simulink subsystem "PvtSubSys_LATC"  (R2020b)
settings: Solver=VariableStepAuto  StartTime=0.0  StopTime=10.0  RelTol=1e-3
undefined symbols (not defined in the file or in its folder): LCS_PLAN_PreViewIdxNum, LCS_PLAN_PreViewIdxSW_b, P_Global_CharSpd_ms, P_Global_SteeringAngleRatio, P_Global_WheelBase_m, P_LCS_DetNoOverRide_DrvTrq_TH, P_LCS_DetOverRide_DrvTrq_TH, P_LCS_ESS_AngleSlope_Limit, P_LCS_ESS_LogicTest_Enable, P_LCS_ESS_NotActiveFlgDelayTime, P_LCS_ESS_NotActiveFlgDelayTimeSW, P_LCS_ESS_SteerAngleErr, P_LCS_ESS_SteerAngleFilterTime, P_LCS_ESS_TarAngleFilterTime, P_LCS_ESSAngleSW, P_LCS_ESSOverrideTime1, P_LCS_ESSOverrideTime2, P_LCS_ESSOverrideTime3, P_LCS_ESSOverrideValue1, P_LCS_ESSOverrideValue2, P_LCS_IN_Offset_Test_SW, P_LCS_IN_Offset_Test_Value, P_LCS_LATC_AngleFilterTime_s, P_LCS_LATC_CurOffsetCurve_TabX_m, P_LCS_LATC_CurOffsetCurveFliterTime_Tab_s, P_LCS_LATC_CurOffsetVehicleSpdLimitValue_degs, P_LCS_LATC_DeltaEps_Tab_s, P_LCS_LATC_DxOffset_Sw, P_LCS_LATC_ELKAngleSlope_ratio, P_LCS_LATC_ELKMaxLatAcc_ms2, P_LCS_LATC_ESSA0Dis_TabX_m, P_LCS_LATC_ESSAddAngleSlope_Tab_degs, P_LCS_LATC_ESSAESAngleSlope_Tab_degs, P_LCS_LATC_ESSAngleSlope_ratio, P_LCS_LATC_ESSMaxLatAcc_ms2, P_LCS_LATC_LCAngleSlope_ratio, P_LCS_LATC_LCAngleSlope_Tab_degs, P_LCS_LATC_LCCancleMaxLatAcc_ms2, P_LCS_LATC_LCEcoAngleSlope_ratio, P_LCS_LATC_LCEcoAngleSlope_Tab_degs, P_LCS_LATC_LCEcoMaxLatAcc_ms2, P_LCS_LATC_LCKAngleSlope_ratio, P_LCS_LATC_LCKAngleSlope_Tab_degs, P_LCS_LATC_LCKIEAngleSlope_ratio, P_LCS_LATC_LCKIEAngleSlope_Tab_degs, P_LCS_LATC_LCKIEMaxLatAcc_ms2, P_LCS_LATC_LCKMaxLatAcc_ms2, P_LCS_LATC_LCNormalAngleSlope_ratio, P_LCS_LATC_LCNormalAngleSlope_Tab_degs, P_LCS_LATC_LCNormalMaxLatAcc_ms2, P_LCS_LATC_LCSportAngleSlope_ratio, P_LCS_LATC_LCSportAngleSlope_Tab_degs, P_LCS_LATC_LCSportMaxLatAcc_ms2, P_LCS_LATC_LKAAngleSlope_ratio, P_LCS_LATC_LKAAngleSlope_Tab_degs, P_LCS_LATC_LKAMaxLatAcc_ms2, P_LCS_LATC_MatrixQ1_st, P_LCS_LATC_MatrixQ3_st, P_LCS_LATC_MatrixR_st, P_LCS_LATC_MPCDeltaT_s ... (+70)
libraries: simulink x34
(part 4 of 5)

== system PvtSubSys_LATC/Subsystem/LateralControl/LCS_Angle/Lateral_Control/Dynamic_Model_LQR/SteerAngSlopeCalc/Switch Case Action Subsystem ==
  Flg : Inport
  StateHoldTime : Inport  Port=2
  Action Port : ActionPort
  LC_start_slope : Lookup_n-D  BreakpointsForDimension1=P_LCS_LATC_StateActiveFlg_TabX_st  BreakpointsForDimension2=P_LCS_LATC_StateActiveHoldTime_TabY_st  Table=P_LCS_LATC_StateActivAngleSlopeLimit_ratio  ExtrapMethod=Clip  UseLastTableValue=on  InternalRulePriority=Speed  OutDataTypeStr=single  RndMeth=Simplest
      settings: InputPortMap=u0,u1
  Out1 : Outport
  wires:
  Flg/1 -> LC_start_slope/1
  LC_start_slope/1 -> Out1/1
  StateHoldTime/1 -> LC_start_slope/2

== system PvtSubSys_LATC/Subsystem/LateralControl/LCS_Angle/Lateral_Control/Dynamic_Model_LQR/SteerAngSlopeCalc/Switch Case Action Subsystem1 ==
  Action Port : ActionPort
  Constant : Constant  Value=100  OutDataTypeStr=single
  Out1 : Outport
  wires:
  Constant/1 -> Out1/1

== system PvtSubSys_LATC/Subsystem/LateralControl/LCS_Angle/Lateral_Control/Dynamic_Model_LQR/Understeer&Offset_Calc/Enabled Subsystem ==
  AckConst : Inport
  Raw : Inport  Port=2
  Curve : Inport  Port=3
  Enable : EnablePort
  Constant2 : Constant  Value=0.02  OutDataTypeStr=single
  Constant7 : Constant  Value=P_Global_SteeringAngleRatio
  Constant8 : Constant  Value=57.3  OutDataTypeStr=single
  FilterTime2 : Product  Inputs=4  RndMeth=Zero
  Product2 : Product  Inputs=*/  RndMeth=Zero
  Product6 : Product  RndMeth=Zero
  Sum6 : Sum  Inputs=+-
  Sum7 : Sum
  Unit Delay : UnitDelay  SampleTime=-1  HasFrameUpgradeWarning=on
  predis_ayFac1 : Lookup_n-D  NumberOfTableDimensions=1  BreakpointsForDimension1=P_LCS_LATC_CurOffsetCurve_TabX_m  Table=P_LCS_LATC_CurOffsetCurveFliterTime_Tab_s  ExtrapMethod=Clip  UseLastTableValue=on  InternalRulePriority=Speed  RndMeth=Simplest  InputSameDT=on
  SteerAngleOffset_deg : Outport
  wires:
  Sum7/1 -> SteerAngleOffset_deg/1, Unit Delay/1
  Unit Delay/1 -> Sum6/2, Sum7/2
  Constant2/1 -> Product2/1
  Sum6/1 -> Product6/2
  Product2/1 -> Product6/1
  Product6/1 -> Sum7/1
  Constant7/1 -> FilterTime2/1
  Constant8/1 -> FilterTime2/2
  AckConst/1 -> FilterTime2/3
  Raw/1 -> FilterTime2/4
  FilterTime2/1 -> Sum6/1
  Curve/1 -> predis_ayFac1/1
  predis_ayFac1/1 -> Product2/2

== system PvtSubSys_LATC/Subsystem/LateralControl/LCS_Angle/Lateral_Control/MPC/TargetSteerAngleCalc/LP filter ==
  Raw : Inport
  TorqFilterTime : Inport  Port=2
  Product1 : Product  RndMeth=Zero
  Product4 : Product  Inputs=*/  RndMeth=Zero
  Sum4 : Sum  Inputs=+-|
  Sum5 : Sum
  Unit Delay : UnitDelay  SampleTime=-1  HasFrameUpgradeWarning=on
  Weight/N3 : Constant  Value=0.02  OutDataTypeStr=single
  output : Outport
  wires:
  Sum5/1 -> output/1, Unit Delay/1
  Unit Delay/1 -> Sum5/2, Sum4/2
  Sum4/1 -> Product1/2
  Product1/1 -> Sum5/1
  Raw/1 -> Sum4/1
  Weight/N3/1 -> Product4/1
  Product4/1 -> Product1/1
  TorqFilterTime/1 -> Product4/2

== system PvtSubSys_LATC/Subsystem/LateralControl/LCS_Angle/Lateral_Control/MPC/TargetSteerAngleCalc/LP filter1 ==
  Raw : Inport
  TorqFilterTime : Inport  Port=2
  Memory2 : Memory  InheritSampleTime=on
  Product1 : Product  RndMeth=Zero
  Product4 : Product  Inputs=*/  RndMeth=Zero
  Sum4 : Sum  Inputs=+-|
  Sum5 : Sum  Inputs=++|
  Weight/N3 : Constant  Value=0.02  OutDataTypeStr=single
  output : Outport
  wires:
  TorqFilterTime/1 -> Product4/2
  Product4/1 -> Product1/1
  Weight/N3/1 -> Product4/1
  Raw/1 -> Sum4/1
  Product1/1 -> Sum5/1
  Sum4/1 -> Product1/2
  Memory2/1 -> Sum4/2, Sum5/2
  Sum5/1 -> output/1, Memory2/1

== system PvtSubSys_LATC/Subsystem/LateralControl/LCS_Angle/Lateral_Control/MPC/TargetSteerAngleCalc/Subsystem ==
  Flg : Inport
  HoldTime : Inport  Port=2
  Merge : Merge
  Merge1 : Merge
  Merge2 : Merge
  Switch Case : SwitchCase  CaseConditions={[1,2,3,4,5]}
  Switch Case Action Subsystem : Subsystem  TreatAsAtomicUnit=on
  Switch Case Action Subsystem1 : Subsystem  TreatAsAtomicUnit=on
  Switch Case Action Subsystem2 : Subsystem  TreatAsAtomicUnit=on
  Switch Case Action Subsystem3 : Subsystem  TreatAsAtomicUnit=on
  Switch Case Action Subsystem4 : Subsystem  TreatAsAtomicUnit=on
  Switch Case Action Subsystem5 : Subsystem  TreatAsAtomicUnit=on
  Switch Case1 : SwitchCase  CaseConditions={[6,7,8]}
  Switch Case2 : SwitchCase  CaseConditions={[6,7,8]}
  LC_Complete_AngleSlope : Outport
  LC_Complete_PreDisFac : Outport  Port=2
  StateActiv_AngleSlope : Outport  Port=3
  wires:
  [HoldTime] -> Switch Case Action Subsystem2/2(StateHoldTime)
  Switch Case/2 -> Switch Case Action Subsystem1/Action
  Switch Case Action Subsystem4/1(Out1) -> Merge2/1
  Switch Case Action Subsystem1/1(Out1) -> Merge/1
  Switch Case Action Subsystem3/1(Out1) -> Merge1/1
  Switch Case2/2 -> Switch Case Action Subsystem4/Action
  HoldTime/1 -> Switch Case Action Subsystem5/2(StateHoldTime)
  Flg/1 -> Switch Case/1, Switch Case1/1, Switch Case Action Subsystem5/1(Flg), Switch Case2/1, Switch Case Action Subsystem2/1(Flg), Switch Case Action Subsystem/1(Flg)
  Switch Case2/1 -> Switch Case Action Subsystem5/Action
  Switch Case1/2 -> Switch Case Action Subsystem3/Action
  Switch Case1/1 -> Switch Case Action Subsystem2/Action
  Switch Case Action Subsystem/1(Out1) -> Merge/2
  Switch Case Action Subsystem2/1(Out1) -> Merge1/2
  Switch Case Action Subsystem5/1(LC_Complete_PreDisFac) -> Merge2/2
  Merge2/1 -> LC_Complete_PreDisFac/1
  [HoldTime] -> Switch Case Action Subsystem/2(StateHoldTime)
  Switch Case/1 -> Switch Case Action Subsystem/Action
  Merge1/1 -> LC_Complete_AngleSlope/1
  Merge/1 -> StateActiv_AngleSlope/1

== system PvtSubSys_LATC/Subsystem/LateralControl/LCS_Angle/Lateral_Control/MPC/Understeer_Offset_Calc/Enabled Subsystem ==
  AckConst : Inport
  Raw : Inport  Port=2
  Curve : Inport  Port=3
  Enable : EnablePort
  Constant2 : Constant  Value=0.02  OutDataTypeStr=single
  Constant7 : Constant  Value=P_Global_SteeringAngleRatio
  Constant8 : Constant  Value=57.3  OutDataTypeStr=single
  FilterTime2 : Product  Inputs=4  RndMeth=Zero
  Product2 : Product  Inputs=*/  RndMeth=Zero
  Product6 : Product  RndMeth=Zero
  Sum6 : Sum  Inputs=+-
  Sum7 : Sum
  Unit Delay : UnitDelay  SampleTime=-1  HasFrameUpgradeWarning=on
  predis_ayFac1 : Lookup_n-D  NumberOfTableDimensions=1  BreakpointsForDimension1=P_LCS_LATC_CurOffsetCurve_TabX_m  Table=P_LCS_LATC_CurOffsetCurveFliterTime_Tab_s  ExtrapMethod=Clip  UseLastTableValue=on  InternalRulePriority=Speed  RndMeth=Simplest  InputSameDT=on
  SteerAngleOffset_deg : Outport
  wires:
  Sum7/1 -> SteerAngleOffset_deg/1, Unit Delay/1
  Unit Delay/1 -> Sum6/2, Sum7/2
  Constant2/1 -> Product2/1
  Sum6/1 -> Product6/2
  Product2/1 -> Product6/1
  Product6/1 -> Sum7/1
  Constant7/1 -> FilterTime2/1
  Constant8/1 -> FilterTime2/2
  AckConst/1 -> FilterTime2/3
  Raw/1 -> FilterTime2/4
  FilterTime2/1 -> Sum6/1
  Curve/1 -> predis_ayFac1/1
  predis_ayFac1/1 -> Product2/2

== system PvtSubSys_LATC/Subsystem/LateralControl/LCS_Angle/Lateral_Control/kinematics_MPC/SteerAngSlopeCalc/Switch Case Action Subsystem ==
  Flg : Inport
  StateHoldTime : Inport  Port=2
  Action Port : ActionPort
  LC_start_slope : Lookup_n-D  BreakpointsForDimension1=P_LCS_LATC_StateActiveFlg_TabX_st  BreakpointsForDimension2=P_LCS_LATC_StateActiveHoldTime_TabY_st  Table=P_LCS_LATC_StateActivAngleSlopeLimit_ratio  ExtrapMethod=Clip  UseLastTableValue=on  InternalRulePriority=Speed  OutDataTypeStr=single  RndMeth=Simplest
      settings: InputPortMap=u0,u1
  Out1 : Outport
  wires:
  Flg/1 -> LC_start_slope/1
  LC_start_slope/1 -> Out1/1
  StateHoldTime/1 -> LC_start_slope/2

== system PvtSubSys_LATC/Subsystem/LateralControl/LCS_Angle/Lateral_Control/kinematics_MPC/SteerAngSlopeCalc/Switch Case Action Subsystem1 ==
  Action Port : ActionPort
  Constant : Constant  Value=100  OutDataTypeStr=single
  Out1 : Outport
  wires:
  Constant/1 -> Out1/1

== system PvtSubSys_LATC/Subsystem/LateralControl/LCS_Angle/Lateral_Control/kinematics_MPC/Understeer&Offset_Calc/Enabled Subsystem ==
  AckConst : Inport
  Raw : Inport  Port=2
  Curve : Inport  Port=3
  Enable : EnablePort
  Constant2 : Constant  Value=0.02  OutDataTypeStr=single
  Constant7 : Constant  Value=P_Global_SteeringAngleRatio
  Constant8 : Constant  Value=57.3  OutDataTypeStr=single
  FilterTime2 : Product  Inputs=4  RndMeth=Zero
  Product2 : Product  Inputs=*/  RndMeth=Zero
  Product6 : Product  RndMeth=Zero
  Sum6 : Sum  Inputs=+-
  Sum7 : Sum
  Unit Delay : UnitDelay  SampleTime=-1  HasFrameUpgradeWarning=on
  predis_ayFac1 : Lookup_n-D  NumberOfTableDimensions=1  BreakpointsForDimension1=P_LCS_LATC_CurOffsetCurve_TabX_m  Table=P_LCS_LATC_CurOffsetCurveFliterTime_Tab_s  ExtrapMethod=Clip  UseLastTableValue=on  InternalRulePriority=Speed  RndMeth=Simplest  InputSameDT=on
  SteerAngleOffset_deg : Outport
  wires:
  Sum7/1 -> SteerAngleOffset_deg/1, Unit Delay/1
  Unit Delay/1 -> Sum6/2, Sum7/2
  Constant2/1 -> Product2/1
  Sum6/1 -> Product6/2
  Product2/1 -> Product6/1
  Product6/1 -> Sum7/1
  Constant7/1 -> FilterTime2/1
  Constant8/1 -> FilterTime2/2
  AckConst/1 -> FilterTime2/3
  Raw/1 -> FilterTime2/4
  FilterTime2/1 -> Sum6/1
  Curve/1 -> predis_ayFac1/1
  predis_ayFac1/1 -> Product2/2

== system PvtSubSys_LATC/Subsystem/LateralControl/LCS_Angle/Motion_Planning/CartesianTrajectory/Subsystem1/LP filter ==
  Raw : Inport
  TorqFilterTime : Inport  Port=2
  Product1 : Product  RndMeth=Zero
  Product4 : Product  Inputs=*/  RndMeth=Zero
  Sum4 : Sum  Inputs=+-
  Sum5 : Sum
  Unit Delay : UnitDelay  SampleTime=-1  HasFrameUpgradeWarning=on
  Weight/N3 : Constant  Value=0.02  OutDataTypeStr=single
  output : Outport
  wires:
  Sum5/1 -> output/1, Unit Delay/1
  Unit Delay/1 -> Sum5/2, Sum4/2
  Sum4/1 -> Product1/2
  Product1/1 -> Sum5/1
  Raw/1 -> Sum4/1
  Weight/N3/1 -> Product4/1
  Product4/1 -> Product1/1
  TorqFilterTime/1 -> Product4/2

== system PvtSubSys_LATC/Subsystem/LateralControl/LCS_Angle/Motion_Planning/CartesianTrajectory/Subsystem1/Switch Case Action Subsystem ==
  Flg : Inport
  StateHoldTime : Inport  Port=2
  Action Port : ActionPort
  ActiveAyDtLimit_TBL : Lookup_n-D  BreakpointsForDimension1=P_LCS_LATC_StateActiveFlg_TabX_st  BreakpointsForDimension2=P_LCS_LATC_StateActiveHoldTime_TabY_st  Table=P_LCS_PLAN_StateActiv_AyDtLimit_ms3  ExtrapMethod=Clip  UseLastTableValue=on  InternalRulePriority=Speed  OutDataTypeStr=single  RndMeth=Simplest
      settings: InputPortMap=u0,u1
  ActivePreviewT_TBL : Lookup_n-D  BreakpointsForDimension1=P_LCS_LATC_StateActiveFlg_TabX_st  BreakpointsForDimension2=P_LCS_LATC_StateActiveHoldTime_TabY_st  Table=P_LCS_PLAN_StateActiv_PreviewT_s  ExtrapMethod=Clip  UseLastTableValue=on  InternalRulePriority=Speed  OutDataTypeStr=single  RndMeth=Simplest
      settings: InputPortMap=u0,u1
  PreviewT : Outport
  AyDtLimit : Outport  Port=2
  wires:
  StateHoldTime/1 -> ActiveAyDtLimit_TBL/2, ActivePreviewT_TBL/2
  ActivePreviewT_TBL/1 -> PreviewT/1
  Flg/1 -> ActiveAyDtLimit_TBL/1, ActivePreviewT_TBL/1
  ActiveAyDtLimit_TBL/1 -> AyDtLimit/1

== system PvtSubSys_LATC/Subsystem/LateralControl/LCS_Angle/Motion_Planning/CartesianTrajectory/Subsystem1/Switch Case Action Subsystem1 ==
  Action Port : ActionPort
  Constant : Constant  Value=100  OutDataTypeStr=single
  Constant1 : Constant  Value=100  OutDataTypeStr=single
  PreviewT : Outport
  AyDtLimit : Outport  Port=2
  wires:
  Constant/1 -> PreviewT/1
  Constant1/1 -> AyDtLimit/1

== system PvtSubSys_LATC/Subsystem/LateralControl/LCS_Angle/Motion_Planning/CartesianTrajectory_MPC/Subsystem/LP filter ==
  Raw : Inport
  TorqFilterTime : Inport  Port=2
  Memory2 : Memory  InheritSampleTime=on
  Product1 : Product  RndMeth=Zero
  Product4 : Product  Inputs=*/  RndMeth=Zero
  Sum4 : Sum  Inputs=+-|
  Sum5 : Sum  Inputs=++|
  Weight/N3 : Constant  Value=0.02  OutDataTypeStr=single
  output : Outport
  wires:
  TorqFilterTime/1 -> Product4/2
  Product4/1 -> Product1/1
  Weight/N3/1 -> Product4/1
  Raw/1 -> Sum4/1
  Product1/1 -> Sum5/1
  Sum4/1 -> Product1/2
  Memory2/1 -> Sum4/2, Sum5/2
  Sum5/1 -> output/1, Memory2/1

== system PvtSubSys_LATC/Subsystem/LateralControl/LCS_Angle/Motion_Planning/CartesianTrajectory_MPC/Subsystem/Subsystem ==
  Flg : Inport
  HoldTime : Inport  Port=2
  Merge : Merge
  Merge1 : Merge
  Merge2 : Merge
  Switch Case : SwitchCase  CaseConditions={[1,2,3,4,5]}
  Switch Case Action Subsystem : Subsystem  TreatAsAtomicUnit=on
  Switch Case Action Subsystem1 : Subsystem  TreatAsAtomicUnit=on
  Switch Case Action Subsystem2 : Subsystem  TreatAsAtomicUnit=on
  Switch Case Action Subsystem3 : Subsystem  TreatAsAtomicUnit=on
  Switch Case Action Subsystem4 : Subsystem  TreatAsAtomicUnit=on
  Switch Case Action Subsystem5 : Subsystem  TreatAsAtomicUnit=on
  Switch Case1 : SwitchCase  CaseConditions={[6,7,8]}
  Switch Case2 : SwitchCase  CaseConditions={[6,7,8]}
  LC_Complete_AngleSlope : Outport
  LC_Complete_PreDisFac : Outport  Port=2
  StateActiv_AngleSlope : Outport  Port=3
  wires:
  [HoldTime] -> Switch Case Action Subsystem2/2(StateHoldTime)
  Switch Case/2 -> Switch Case Action Subsystem1/Action
  Switch Case Action Subsystem4/1(Out1) -> Merge2/1
  Switch Case Action Subsystem1/1(Out1) -> Merge/1
  Switch Case Action Subsystem3/1(Out1) -> Merge1/1
  Switch Case2/2 -> Switch Case Action Subsystem4/Action
  HoldTime/1 -> Switch Case Action Subsystem5/2(StateHoldTime)
  Flg/1 -> Switch Case/1, Switch Case1/1, Switch Case Action Subsystem5/1(Flg), Switch Case2/1, Switch Case Action Subsystem2/1(Flg), Switch Case Action Subsystem/1(Flg)
  Switch Case2/1 -> Switch Case Action Subsystem5/Action
  Switch Case1/2 -> Switch Case Action Subsystem3/Action
  Switch Case1/1 -> Switch Case Action Subsystem2/Action
  Switch Case Action Subsystem/1(Out1) -> Merge/2
  Switch Case Action Subsystem2/1(Out1) -> Merge1/2
  Switch Case Action Subsystem5/1(LC_Complete_PreDisFac) -> Merge2/2
  Merge2/1 -> LC_Complete_PreDisFac/1
  [HoldTime] -> Switch Case Action Subsystem/2(StateHoldTime)
  Switch Case/1 -> Switch Case Action Subsystem/Action
  Merge1/1 -> LC_Complete_AngleSlope/1
  Merge/1 -> StateActiv_AngleSlope/1

== system PvtSubSys_LATC/Subsystem/LateralControl/LCS_Angle/Motion_Planning/FrenetTrajectory/Subsystem/LP filter ==
  Raw : Inport
  TorqFilterTime : Inport  Port=2
  Product1 : Product  RndMeth=Zero
  Product4 : Product  Inputs=*/  RndMeth=Zero
  Sum4 : Sum  Inputs=+-
  Sum5 : Sum
  Unit Delay : UnitDelay  SampleTime=-1  HasFrameUpgradeWarning=on
  Weight/N3 : Constant  Value=0.02  OutDataTypeStr=single
  output : Outport
  wires:
  Sum5/1 -> output/1, Unit Delay/1
  Unit Delay/1 -> Sum5/2, Sum4/2
  Sum4/1 -> Product1/2
  Product1/1 -> Sum5/1
  Raw/1 -> Sum4/1
  Weight/N3/1 -> Product4/1
  Product4/1 -> Product1/1
  TorqFilterTime/1 -> Product4/2

== system PvtSubSys_LATC/Subsystem/LateralControl/LCS_Angle/Motion_Planning/FrenetTrajectory/Subsystem/Switch Case Action Subsystem ==
  Flg : Inport
  StateHoldTime : Inport  Port=2
  Action Port : ActionPort
  ActiveAyDtLimit_TBL : Lookup_n-D  BreakpointsForDimension1=P_LCS_LATC_StateActiveFlg_TabX_st  BreakpointsForDimension2=P_LCS_LATC_StateActiveHoldTime_TabY_st  Table=P_LCS_PLAN_StateActiv_AyDtLimit_ms3  ExtrapMethod=Clip  UseLastTableValue=on  InternalRulePriority=Speed  OutDataTypeStr=single  RndMeth=Simplest
      settings: InputPortMap=u0,u1
  ActivePreviewT_TBL : Lookup_n-D  BreakpointsForDimension1=P_LCS_LATC_StateActiveFlg_TabX_st  BreakpointsForDimension2=P_LCS_LATC_StateActiveHoldTime_TabY_st  Table=P_LCS_PLAN_StateActiv_PreviewT_s  ExtrapMethod=Clip  UseLastTableValue=on  InternalRulePriority=Speed  OutDataTypeStr=single  RndMeth=Simplest
      settings: InputPortMap=u0,u1
  PreviewT : Outport
  AyDtLimit : Outport  Port=2
  wires:
  StateHoldTime/1 -> ActiveAyDtLimit_TBL/2, ActivePreviewT_TBL/2
  ActivePreviewT_TBL/1 -> PreviewT/1
  Flg/1 -> ActiveAyDtLimit_TBL/1, ActivePreviewT_TBL/1
  ActiveAyDtLimit_TBL/1 -> AyDtLimit/1

== system PvtSubSys_LATC/Subsystem/LateralControl/LCS_Angle/Motion_Planning/FrenetTrajectory/Subsystem/Switch Case Action Subsystem1 ==
  Action Port : ActionPort
  Constant : Constant  Value=100  OutDataTypeStr=single
  Constant1 : Constant  Value=100  OutDataTypeStr=single
  PreviewT : Outport
  AyDtLimit : Outport  Port=2
  wires:
  Constant/1 -> PreviewT/1
  Constant1/1 -> AyDtLimit/1

== system PvtSubSys_LATC/Subsystem/LateralControl/LCS_Angle/Motion_Planning/FrenetTrajectory_Lateral/Subsystem1/LP filter ==
  Raw : Inport
  TorqFilterTime : Inport  Port=2
  Product1 : Product  RndMeth=Zero
  Product4 : Product  Inputs=*/  RndMeth=Zero
  Sum4 : Sum  Inputs=+-
  Sum5 : Sum
  Unit Delay : UnitDelay  SampleTime=-1  HasFrameUpgradeWarning=on
  Weight/N3 : Constant  Value=0.02  OutDataTypeStr=single
  output : Outport
  wires:
  Sum5/1 -> output/1, Unit Delay/1
  Unit Delay/1 -> Sum5/2, Sum4/2
  Sum4/1 -> Product1/2
  Product1/1 -> Sum5/1
  Raw/1 -> Sum4/1
  Weight/N3/1 -> Product4/1
  Product4/1 -> Product1/1
  TorqFilterTime/1 -> Product4/2

== system PvtSubSys_LATC/Subsystem/LateralControl/LCS_Angle/Motion_Planning/FrenetTrajectory_Lateral/Subsystem1/Switch Case Action Subsystem ==
  Flg : Inport
  StateHoldTime : Inport  Port=2
  Action Port : ActionPort
  ActiveAyDtLimit_TBL : Lookup_n-D  BreakpointsForDimension1=P_LCS_LATC_StateActiveFlg_TabX_st  BreakpointsForDimension2=P_LCS_LATC_StateActiveHoldTime_TabY_st  Table=P_LCS_PLAN_StateActiv_AyDtLimit_ms3  ExtrapMethod=Clip  UseLastTableValue=on  InternalRulePriority=Speed  OutDataTypeStr=single  RndMeth=Simplest
      settings: InputPortMap=u0,u1
  ActivePreviewT_TBL : Lookup_n-D  BreakpointsForDimension1=P_LCS_LATC_StateActiveFlg_TabX_st  BreakpointsForDimension2=P_LCS_LATC_StateActiveHoldTime_TabY_st  Table=P_LCS_PLAN_StateActiv_PreviewT_s  ExtrapMethod=Clip  UseLastTableValue=on  InternalRulePriority=Speed  OutDataTypeStr=single  RndMeth=Simplest
      settings: InputPortMap=u0,u1
  PreviewT : Outport
  AyDtLimit : Outport  Port=2
  wires:
  StateHoldTime/1 -> ActiveAyDtLimit_TBL/2, ActivePreviewT_TBL/2
  ActivePreviewT_TBL/1 -> PreviewT/1
  Flg/1 -> ActiveAyDtLimit_TBL/1, ActivePreviewT_TBL/1
  ActiveAyDtLimit_TBL/1 -> AyDtLimit/1

== system PvtSubSys_LATC/Subsystem/LateralControl/LCS_Angle/Motion_Planning/FrenetTrajectory_Lateral/Subsystem1/Switch Case Action Subsystem1 ==
  Action Port : ActionPort
  Constant : Constant  Value=100  OutDataTypeStr=single
  Constant1 : Constant  Value=100  OutDataTypeStr=single
  PreviewT : Outport
  AyDtLimit : Outport  Port=2
  wires:
  Constant/1 -> PreviewT/1
  Constant1/1 -> AyDtLimit/1

== system PvtSubSys_LATC/Subsystem/LateralControl/LCS_Angle/Lateral_Control/MPC/TargetSteerAngleCalc/Subsystem/Switch Case Action Subsystem ==
  Flg : Inport
  StateHoldTime : Inport  Port=2
  Action Port : ActionPort
  LC_start_slope : Lookup_n-D  BreakpointsForDimension1=P_LCS_PLAN_StateActiveFlg_TabX_st  BreakpointsForDimension2=P_LCS_PLAN_StateActiveHoldTime_TabY_s  Table=P_LCS_PLAN_StateActivAngleSlope_Tab_ratio  ExtrapMethod=Clip  UseLastTableValue=on  InternalRulePriority=Speed  OutDataTypeStr=single  RndMeth=Simplest
      settings: InputPortMap=u0,u1
  Out1 : Outport
  wires:
  Flg/1 -> LC_start_slope/1
  LC_start_slope/1 -> Out1/1
  StateHoldTime/1 -> LC_start_slope/2

== system PvtSubSys_LATC/Subsystem/LateralControl/LCS_Angle/Lateral_Control/MPC/TargetSteerAngleCalc/Subsystem/Switch Case Action Subsystem1 ==
  Action Port : ActionPort
  Constant : Constant  Value=100  OutDataTypeStr=single
  Out1 : Outport
  wires:
  Constant/1 -> Out1/1

== system PvtSubSys_LATC/Subsystem/LateralControl/LCS_Angle/Lateral_Control/MPC/TargetSteerAngleCalc/Subsystem/Switch Case Action Subsystem2 ==
  Flg : Inport
  StateHoldTime : Inport  Port=2
  Action Port : ActionPort
  LC_start_slope : Lookup_n-D  BreakpointsForDimension1=P_LCS_PLAN_StateCompleteFlg_TabX_st  BreakpointsForDimension2=P_LCS_PLAN_StateActiveHoldTime_TabY_s  Table=P_LCS_PLAN_StateCompleteAngleSlope_Tab_ratio  ExtrapMethod=Clip  UseLastTableValue=on  InternalRulePriority=Speed  OutDataTypeStr=single  RndMeth=Simplest
      settings: InputPortMap=u0,u1
  Out1 : Outport
  wires:
  StateHoldTime/1 -> LC_start_slope/2
  LC_start_slope/1 -> Out1/1
  Flg/1 -> LC_start_slope/1

== system PvtSubSys_LATC/Subsystem/LateralControl/LCS_Angle/Lateral_Control/MPC/TargetSteerAngleCalc/Subsystem/Switch Case Action Subsystem3 ==
  Action Port : ActionPort
  Constant : Constant  Value=0.3  OutDataTypeStr=single
  Out1 : Outport
  wires:
  Constant/1 -> Out1/1

== system PvtSubSys_LATC/Subsystem/LateralControl/LCS_Angle/Lateral_Control/MPC/TargetSteerAngleCalc/Subsystem/Switch Case Action Subsystem4 ==
  Action Port : ActionPort
  Constant : Constant  OutDataTypeStr=single
  Out1 : Outport
  wires:
  Constant/1 -> Out1/1

== system PvtSubSys_LATC/Subsystem/LateralControl/LCS_Angle/Lateral_Control/MPC/TargetSteerAngleCalc/Subsystem/Switch Case Action Subsystem5 ==
  Flg : Inport
  StateHoldTime : Inport  Port=2
  Action Port : ActionPort
  LC_start_slope : Lookup_n-D  BreakpointsForDimension1=P_LCS_PLAN_StateCompleteFlg_TabX_st  BreakpointsForDimension2=P_LCS_PLAN_StateActiveHoldTime_TabY_s  Table=P_LCS_PLAN_LCCompletePreDisFac_Tab_ratio  ExtrapMethod=Clip  UseLastTableValue=on  InternalRulePriority=Speed  OutDataTypeStr=single  RndMeth=Simplest
      settings: InputPortMap=u0,u1
  LC_Complete_PreDisFac : Outport
  wires:
  Flg/1 -> LC_start_slope/1
  LC_start_slope/1 -> LC_Complete_PreDisFac/1
  StateHoldTime/1 -> LC_start_slope/2

== system PvtSubSys_LATC/Subsystem/LateralControl/LCS_Angle/Motion_Planning/CartesianTrajectory_MPC/Subsystem/Subsystem/Switch Case Action Subsystem ==
  Flg : Inport
  StateHoldTime : Inport  Port=2
  Action Port : ActionPort
  LC_start_slope : Lookup_n-D  BreakpointsForDimension1=P_LCS_PLAN_StateActiveFlg_TabX_st  BreakpointsForDimension2=P_LCS_PLAN_StateActiveHoldTime_TabY_s  Table=P_LCS_PLAN_StateActivAngleSlope_Tab_ratio  ExtrapMethod=Clip  UseLastTableValue=on  InternalRulePriority=Speed  OutDataTypeStr=single  RndMeth=Simplest
      settings: InputPortMap=u0,u1
  Out1 : Outport
  wires:
  Flg/1 -> LC_start_slope/1
  LC_start_slope/1 -> Out1/1
  StateHoldTime/1 -> LC_start_slope/2

== system PvtSubSys_LATC/Subsystem/LateralControl/LCS_Angle/Motion_Planning/CartesianTrajectory_MPC/Subsystem/Subsystem/Switch Case Action Subsystem1 ==
  Action Port : ActionPort
  Constant : Constant  Value=100  OutDataTypeStr=single
  Out1 : Outport
  wires:
  Constant/1 -> Out1/1

== system PvtSubSys_LATC/Subsystem/LateralControl/LCS_Angle/Motion_Planning/CartesianTrajectory_MPC/Subsystem/Subsystem/Switch Case Action Subsystem2 ==
  Flg : Inport
  StateHoldTime : Inport  Port=2
  Action Port : ActionPort
  LC_start_slope : Lookup_n-D  BreakpointsForDimension1=P_LCS_PLAN_StateCompleteFlg_TabX_st  BreakpointsForDimension2=P_LCS_PLAN_StateActiveHoldTime_TabY_s  Table=P_LCS_PLAN_StateCompleteAngleSlope_Tab_ratio  ExtrapMethod=Clip  UseLastTableValue=on  InternalRulePriority=Speed  OutDataTypeStr=single  RndMeth=Simplest
      settings: InputPortMap=u0,u1
  Out1 : Outport
  wires:
  StateHoldTime/1 -> LC_start_slope/2
  LC_start_slope/1 -> Out1/1
  Flg/1 -> LC_start_slope/1

== system PvtSubSys_LATC/Subsystem/LateralControl/LCS_Angle/Motion_Planning/CartesianTrajectory_MPC/Subsystem/Subsystem/Switch Case Action Subsystem3 ==
  Action Port : ActionPort
  Constant : Constant  Value=0.3  OutDataTypeStr=single
  Out1 : Outport
  wires:
  Constant/1 -> Out1/1

== system PvtSubSys_LATC/Subsystem/LateralControl/LCS_Angle/Motion_Planning/CartesianTrajectory_MPC/Subsystem/Subsystem/Switch Case Action Subsystem4 ==
  Action Port : ActionPort
  Constant : Constant  OutDataTypeStr=single
  Out1 : Outport
  wires:
  Constant/1 -> Out1/1

== system PvtSubSys_LATC/Subsystem/LateralControl/LCS_Angle/Motion_Planning/CartesianTrajectory_MPC/Subsystem/Subsystem/Switch Case Action Subsystem5 ==
  Flg : Inport
  StateHoldTime : Inport  Port=2
  Action Port : ActionPort
  LC_start_slope : Lookup_n-D  BreakpointsForDimension1=P_LCS_PLAN_StateCompleteFlg_TabX_st  BreakpointsForDimension2=P_LCS_PLAN_StateActiveHoldTime_TabY_s  Table=P_LCS_PLAN_LCCompletePreDisFac_Tab_ratio  ExtrapMethod=Clip  UseLastTableValue=on  InternalRulePriority=Speed  OutDataTypeStr=single  RndMeth=Simplest
      settings: InputPortMap=u0,u1
  LC_Complete_PreDisFac : Outport
  wires:
  Flg/1 -> LC_start_slope/1
  LC_start_slope/1 -> LC_Complete_PreDisFac/1
  StateHoldTime/1 -> LC_start_slope/2

== matlab function PvtSubSys_LATC/Subsystem/LateralControl/LCS_Angle/Motion_Planning/FrenetTrajectory_Lateral/FrenetTrajectory_Lateral ==
  data: A0 input; A1 input; A2 input; A3 input; Veh_Speed input size=1; YawRate input size=1; TarDangerlLevel input; PreView_T input size=1; PlanX output; PlanY output; PlanTheta output; idx output; PreviewX output; PreviewY output; PreviewTheta output; numTraj output size=1; ref_curvature output; ref_theta output; AyDtLimit input size=1; Min_Plan_Dis input; lateral_error output size=1; lateral_error_rate output size=1; heading_error output size=1; heading_error_rate output size=1; PreViewIdxSW input; PreViewIdxNum input
function [PlanX,PlanY,PlanTheta,idx,PreviewX,PreviewY,PreviewTheta,numTraj,ref_curvature,ref_theta,lateral_error,lateral_error_rate,heading_error,heading_error_rate] ...
    = FrenetTrajectory_Lateral(A0,A1,A2,A3,Veh_Speed,YawRate,TarDangerlLevel,PreView_T,AyDtLimit,Min_Plan_Dis,PreViewIdxSW,PreViewIdxNum)
Veh_Speed = max(Veh_Speed,2);
%% 参考线离散化
rx1 = [single(0):single(1):single(19)];
rx2 = [single(20):20:150];
rx = cat(2,rx1,rx2);
ry = single((-1)).*(A0 + A1.* rx + A2.* (rx.^2) + A3.* (rx.^3));
waypoints = [ry',rx'];
referencePathPointNum = 100;
referencePath = FrenentReferencePath(waypoints,referencePathPointNum);
pathStart = referencePath.interpolate(0);% 求起始点处车辆状态 [x, y,theta, kappa, dkappa, s]
initialState=[0 -A0 pathStart(1,3)];

Frenet_traj_obj = TrajectoryGeneratorFrenet(referencePath);
FtNumTarpoints = single(40); % Frenet坐标系轨迹点数
GtNumTarpoints = single(40); % 全局坐标系轨迹点数
%% 生成轨迹
Py =single([1.5 2 2.5 3 3.6 4.4 5 5.8 6.4 7	7.8	8.6	9.5 10.4 11.4]);% 按等比1.1
Py = max(Veh_Speed,5) .* Py; % 暂时设定最短规划距离 5*2.5
Px = single((-1)).*(A3.*(Py.^3) + A2.*(Py.^2) + A1.*(Py.^1) + A0);
for i = 1:length(Py)
    arcLenOffsets = 1.05*sqrt(Px(i)^2 + Py(i)^2);
    [frenetTrajectory,globalTrajectory,numTraj] = Frenet_traj_obj.FrenetTrajectory_Lateral(initialState,arcLenOffsets,0,FtNumTarpoints,GtNumTarpoints);
    AyDt = (diff(frenetTrajectory.Trajectory(:,3).*(Veh_Speed*Veh_Speed)))./diff(frenetTrajectory.Trajectory(:,1)./Veh_Speed);
    if all(abs(AyDt(1:end,1)) < AyDtLimit) && (frenetTrajectory.Trajectory(end,1) > Min_Plan_Dis)
        break;
    end
end
numTraj = i;%借用numTraj将第几个时间点输出
[globalTrajectory] = EvaluateTrajectory_Lateral(frenetTrajectory,globalTrajectory, 1,1);
%%
% [s,d]→[x, y, theta, kappa, dkappa]
PlanX = single(zeros(GtNumTarpoints,1));
PlanY = single(zeros(GtNumTarpoints,1));
PlanTheta = single(zeros(GtNumTarpoints,1));
PlanX= globalTrajectory(1).Trajectory(1:GtNumTarpoints,2);
PlanY= globalTrajectory(1).Trajectory(1:GtNumTarpoints,1);
PlanTheta = globalTrajectory(1).Trajectory(1:GtNumTarpoints,3);
[matrix_state,ref_curvature,ref_theta,idx] = Calc_State_Error(Veh_Speed,YawRate,globalTrajectory,PreView_T,GtNumTarpoints,PreViewIdxSW,PreViewIdxNum);
PreviewX = globalTrajectory(1).Trajectory(idx,2);
PreviewY = globalTrajectory(1).Trajectory(idx,1);
PreviewTheta = globalTrajectory(1).Trajectory(idx,3);
% lateral_error = single(zeros(1,1));lateral_error_rate = single(zeros(1,1));heading_error = single(zeros(1,1));heading_error_rate = single(zeros(1,1));
lateral_error = matrix_state(1,1);
lateral_error_rate = matrix_state(2,1);
heading_error = matrix_state(3,1);
heading_error_rate = matrix_state(4,1);

end

== matlab function PvtSubSys_LATC/Subsystem/LateralControl/LCS_Angle/Motion_Planning/CartesianTrajectory_MPC/Subsystem/MATLAB Function3 ==
  data: delytime input uint16; TarDangerLevel input uint8; TarDangerLevelK1 input uint8; FLg output uint8; FLgK1 input uint8; CntK1 input uint16; Cnt output uint16
function [FLg,Cnt] = AngSlopeCalc(delytime,TarDangerLevel,TarDangerLevelK1,FLgK1,CntK1)

Cnt = min(CntK1 + uint16(1),delytime);
if Cnt== delytime
    FLg = uint8(0);
else
    FLg = FLgK1;
end
%FLg = FLgK1;
%% 换道开始检测
if TarDangerLevel==uint8(1) && TarDangerLevelK1==0  % NO function 2 LCK (TarDangerLevelK1==0)
    Cnt =uint16(0);
    FLg = uint8(1);
end
%由LCK状态切换为Normal
if  TarDangerLevel==uint8(3) && (TarDangerLevelK1==uint8(1)||TarDangerLevelK1==uint8(2)) % LCK/IE 2 LC_Normal
    Cnt =uint16(0);
    FLg = uint8(2);
end
%由LCK状态切换为Eco
if  TarDangerLevel==uint8(7) && (TarDangerLevelK1==uint8(1)||TarDangerLevelK1==uint8(2)) % LCK/IE 2 LC_Eco
    Cnt =uint16(0);
    FLg = uint8(3);
end
%由LCK状态切换为Sport
if  TarDangerLevel==uint8(8) && (TarDangerLevelK1==uint8(1)||TarDangerLevelK1==uint8(2)) % LCK/IE 2 LC_sport
    Cnt =uint16(0);
    FLg = uint8(4);
end
if  TarDangerLevel==uint8(6) && (TarDangerLevelK1==uint8(1)||TarDangerLevelK1==uint8(2)) % LCK/IE 2 ESS 后期添加配和ESS Slope 一起调试
    Cnt =uint16(0);
    FLg = uint8(5);
end
%% 换道完成检测，主要时为了解决换道完成后切换到LCK后Angleslope太小导致超调，检测到换道完成后延时一段时间保持一个大斜率。
if  (TarDangerLevel==uint8(1)||TarDangerLevel==uint8(2)) && (TarDangerLevelK1==uint8(3)) % LCK/IE 2 LC_Normal Complete
    Cnt =uint16(0);
    FLg = uint8(6);
end
if  (TarDangerLevel==uint8(1)||TarDangerLevel==uint8(2)) && (TarDangerLevelK1==uint8(7)) % LCK/IE 2 LC_Eco Complete
    Cnt =uint16(0);
    FLg = uint8(7);
end
if  (TarDangerLevel==uint8(1)||TarDangerLevel==uint8(2)) && (TarDangerLevelK1==uint8(8)) % LCK/IE 2 LC_sport Complete
    Cnt =uint16(0);
    FLg = uint8(8);
end

== matlab function PvtSubSys_LATC/Subsystem/LateralControl/LCS_Angle/Motion_Planning/FrenetTrajectory/FrenetTrajectory ==
  data: A0 input; A1 input; A2 input; A3 input; Veh_Speed input size=1; YawRate input size=1; PreView_T input size=1; PlanX output; PlanY output; PlanTheta output; idx output; PreviewX output; PreviewY output; PreviewTheta output; numTraj output size=1; ref_curvature output; ref_theta output; AyDtLimit input size=1; Min_Plan_Dis input; lateral_error output size=1; lateral_error_rate output size=1; heading_error output size=1; heading_error_rate output size=1; PreViewIdxSW input; PreViewIdxNum input
function [PlanX,PlanY,PlanTheta,idx,PreviewX,PreviewY,PreviewTheta,numTraj,ref_curvature,ref_theta,lateral_error,lateral_error_rate,heading_error,heading_error_rate] ...
    = FrenetTrajectory(A0,A1,A2,A3,Veh_Speed,YawRate,PreView_T,AyDtLimit,Min_Plan_Dis,PreViewIdxSW,PreViewIdxNum)
% 参考线离散化
rx1 = [single(0):single(1):single(19)];
rx2 = [single(20):20:150];
rx = cat(2,rx1,rx2);
ry = single((-1)).*(A0 + A1.* rx + A2.* (rx.^2) + A3.* (rx.^3));
waypoints = [ry',rx'];
referencePathPointNum = 100; %参考轨迹的点的个数(参考点的分辨率)，此参数会影响最终目标轨迹线的形状，太小会出现轨迹线拐点
referencePath = FrenentReferencePath(waypoints,referencePathPointNum);
% pathStart = referencePath.interpolate(0);% 求起始点处车辆状态 [x, y,theta, kappa, dkappa, s],车辆在起始点处。%删除此种办法，经过测试发现在弯道或者换道过程中，A1项大的时候轨迹存往反方向突出一点再返回的问题
%% 定义轨迹起始点状态
initGlobalState = [0 0 pi/2 0 Veh_Speed  0]; %暂时定义纵向加速度为0，[x, y,theta, kappa speed，Acc]
initFrenetState = referencePath.global2frenet(initGlobalState);
% Py =single([2.5	2.7	3 3.3 3.6 4 4.4	4.8	5.3	5.8	6.4	7.1	7.8	8.6	9.5 10.4 11.4].*Py_Fac);
Py =single([1.5 2 2.5 3 3.6 4.2 5 5.8 6.4 7	7.8	8.6	9.5 10.4 11.4]);
TarEgoAy = zeros(1,length(Py));% 终点处期望纵向加速度
TarEgoV = ones(1,length(Py)) .* Veh_Speed;% 终点处期望纵向速度
Py = max(Veh_Speed,5).*Py;
Px = single((-1)).*(A3.*(Py.^3) + A2.*(Py.^2) + A1.*(Py.^1) + A0);

Frenet_traj_obj = TrajectoryGeneratorFrenet(referencePath);
FtNumTarpoints = single(40); % Frenet坐标系轨迹点数
%% 生成轨迹
for i = 1:length(Py)
    Pl = round(1.05*sqrt(Px(i)^2 + Py(i)^2));
    Pt = round(1.05*sqrt(Px(i)^2 + Py(i)^2)/max(1,0.5*(TarEgoV(i) + Veh_Speed)));
    pathend= referencePath.interpolate(Pl);
    EndGlobalState = [pathend(1:4) TarEgoV(i) TarEgoAy(i)];
    EndFrenetState = referencePath.global2frenet(EndGlobalState);
    [frenetTrajectory,globalTrajectory] = Frenet_traj_obj.FrenetTrajectory(initFrenetState,EndFrenetState(1,1),0,EndFrenetState(1,2:3),EndFrenetState(1,5:6),Pt,FtNumTarpoints);
    AyDt = abs(diff(globalTrajectory.Trajectory(:,4).*((globalTrajectory.Trajectory(:,5).^2)))./diff(globalTrajectory.Times));
    if all(abs(AyDt)<AyDtLimit) && (frenetTrajectory.Trajectory(end,1) > Min_Plan_Dis)
        break;
    end
end
numTraj  = i;%借用numTraj输出时间点索引号
[globalTrajectory] = EvaluateTrajectory(frenetTrajectory,globalTrajectory,1,1,1,1);
%%
% [s,d]→[x, y, theta, kappa, dkappa]
PlanX = single(zeros(FtNumTarpoints,1));
PlanY = single(zeros(FtNumTarpoints,1));
PlanTheta = single(zeros(FtNumTarpoints,1));
PlanX= globalTrajectory(1).Trajectory(1:FtNumTarpoints,2);
PlanY= globalTrajectory(1).Trajectory(1:FtNumTarpoints,1);
PlanTheta = globalTrajectory(1).Trajectory(1:FtNumTarpoints,3);
[matrix_state,ref_curvature,ref_theta,idx] = Calc_State_Error(Veh_Speed,YawRate,globalTrajectory,PreView_T,FtNumTarpoints,PreViewIdxSW,PreViewIdxNum);
PreviewX = globalTrajectory(1).Trajectory(idx,2);
PreviewY = globalTrajectory(1).Trajectory(idx,1);
PreviewTheta = globalTrajectory(1).Trajectory(idx,3);
% lateral_error = single(zeros(1,1));lateral_error_rate = single(zeros(1,1));heading_error = single(zeros(1,1));heading_error_rate = single(zeros(1,1));
lateral_error = matrix_state(1,1);
lateral_error_rate = matrix_state(2,1);
heading_error = matrix_state(3,1);
heading_error_rate = matrix_state(4,1);

end

== stateflow chart PvtSubSys_LATC/Subsystem/LateralControl/LCS_Angle/OverRideDetect/Chart ==
  state NoOverRide
    en:isOverRide=false;
  state IsOverRide
    en:isOverRide=true;
  (default) -> NoOverRide
  NoOverRide -> IsOverRide : [Ovride]
  IsOverRide -> NoOverRide : [NoOvride]
  data: isOverRide output; Ovride input; NoOvride input

== matlab function PvtSubSys_LATC/Subsystem/LateralControl/LCS_Angle/Motion_Planning/FrenetTrajectory/Subsystem/MATLAB Function ==
  data: Forward_PreViewT input; VehSpd input; PreCurve output; C2 input; C3 input; PreCurve_Abs output
function [PreCurve,PreCurve_Abs]= PreView_Point_Curvature(Forward_PreViewT,VehSpd,C2,C3)
LookForwardDis = VehSpd * Forward_PreViewT;
PreCurve = 6*C3*LookForwardDis + 2*C2;
PreCurve_Abs = abs(PreCurve);
end

== matlab function PvtSubSys_LATC/Subsystem/LateralControl/LCS_Angle/Lateral_Control/MPC/TargetSteerAngleCalc/MATLAB Function3 ==
  data: delytime input uint16; TarDangerLevel input uint8; TarDangerLevelK1 input uint8; FLg output uint8; FLgK1 input uint8; CntK1 input uint16; Cnt output uint16
function [FLg,Cnt] = AngSlopeCalc(delytime,TarDangerLevel,TarDangerLevelK1,FLgK1,CntK1)

Cnt = min(CntK1 + uint16(1),delytime);
if Cnt== delytime
    FLg = uint8(0);
else
    FLg = FLgK1;
end
%FLg = FLgK1;
%% 换道开始检测
if TarDangerLevel==uint8(1) && TarDangerLevelK1==0  % NO function 2 LCK (TarDangerLevelK1==0)
    Cnt =uint16(0);
    FLg = uint8(1);
end
%由LCK状态切换为Normal
if  TarDangerLevel==uint8(3) && (TarDangerLevelK1==uint8(1)||TarDangerLevelK1==uint8(2)) % LCK/IE 2 LC_Normal
    Cnt =uint16(0);
    FLg = uint8(2);
end
%由LCK状态切换为Eco
if  TarDangerLevel==uint8(7) && (TarDangerLevelK1==uint8(1)||TarDangerLevelK1==uint8(2)) % LCK/IE 2 LC_Eco
    Cnt =uint16(0);
    FLg = uint8(3);
end
%由LCK状态切换为Sport
if  TarDangerLevel==uint8(8) && (TarDangerLevelK1==uint8(1)||TarDangerLevelK1==uint8(2)) % LCK/IE 2 LC_sport
    Cnt =uint16(0);
    FLg = uint8(4);
end
if  TarDangerLevel==uint8(6) && (TarDangerLevelK1==uint8(1)||TarDangerLevelK1==uint8(2)) % LCK/IE 2 ESS 后期添加配和ESS Slope 一起调试
    Cnt =uint16(0);
    FLg = uint8(5);
end
%% 换道完成检测，主要时为了解决换道完成后切换到LCK后Angleslope太小导致超调，检测到换道完成后延时一段时间保持一个大斜率。
if  (TarDangerLevel==uint8(1)||TarDangerLevel==uint8(2)) && (TarDangerLevelK1==uint8(3)) % LCK/IE 2 LC_Normal Complete
    Cnt =uint16(0);
    FLg = uint8(6);
end
if  (TarDangerLevel==uint8(1)||TarDangerLevel==uint8(2)) && (TarDangerLevelK1==uint8(7)) % LCK/IE 2 LC_Eco Complete
    Cnt =uint16(0);
    FLg = uint8(7);
end
if  (TarDangerLevel==uint8(1)||TarDangerLevel==uint8(2)) && (TarDangerLevelK1==uint8(8)) % LCK/IE 2 LC_sport Complete
    Cnt =uint16(0);
    FLg = uint8(8);
end

== matlab function PvtSubSys_LATC/Subsystem/LateralControl/LCS_Angle/Motion_Planning/CartesianTrajectory_MPC/CartesianTrajectory ==
  data: planX output single size=11; planY output single size=11; vEgo input size=1; planValid output boolean size=1; kapEgo input size=1; axEgo input size=1; TarLineValid input boolean size=1; TarLineC3 input size=1; TarLineC2 input size=1; TarLineC1 input size=1; TarLineC0 input size=1; ayDtLimit input size=1; planT output; LoopNum output; planLength output; Ay output size=11; AyDt output size=11; break_Flg output; break_AyValue output; break_AyDtValue output; PreDis input; Dis_Fac input; Min_PlanDis input
function [planX,planY,planValid,planT,LoopNum,planLength,Ay,AyDt,break_Flg,break_AyValue,break_AyDtValue] = ...
    linePlanCalc(vEgo, kapEgo,axEgo,...
    TarLineValid,TarLineC3,TarLineC2,TarLineC1,TarLineC0,...
    ayDtLimit,PreDis,Dis_Fac,Min_PlanDis)
%五次多项式规划
LoopNum = 0;
if TarLineValid
    if (abs(TarLineC0)<single(0)) && (abs(TarLineC1)<single(0.05))  %控制线不走中心线，走规划线
        planValid = true;
        planT = single(11);
        planX = single(zeros(11,1));
        planY = single(zeros(11,1));
        planX = single((linspace(0,40,11)))';
        planY = TarLineC3.*planX.^3 + TarLineC2.*planX.^2 + TarLineC1*planX + TarLineC0;
        planLength = planX(end,1);
        Ay = single(zeros(11,1));
        AyDt = single(zeros(11,1));
        break_Flg = uint8(0);
        break_AyValue = single(0);
        break_AyDtValue = single(0);
    else
        Px =single([1.4 1.6 2.1 2.3 2.5 2.7 3 3.3 3.6 4 4.4 4.8 5.3 5.8 6.4 7.1 7.8 8.6 9.5 10.4 11.4]);% 按等比1.1  初选规划时间
        % 定义 TarEgoV、TarEgoAx，由于时间点数变化，导致轨迹条数变化，因此TarEgoV、TarEgoAx维数需要重新定义
        TarEgoAx = zeros(1,length(Px));
        TarEgoV = ones(1,length(Px)) .* vEgo;
        
        if vEgo>single(1)
            Px = vEgo*Px;   %纵向行驶距离
        end
        
        Py = TarLineC3*(Px.^3) + TarLineC2*(Px.^2) + TarLineC1*(Px.^1) + TarLineC0;
        x = single(zeros(11,1));
        y = single(zeros(11,1));
        Vx = single(zeros(11,1));
        Vy = single(zeros(11,1));
        Ax = single(zeros(11,1));
        Ay = single(zeros(11,1));
        AyDt = single(zeros(11,1));
        
        break_Flg = uint8(0);
        break_AyValue = single(0);
        break_AyDtValue = single(0);

        Pt = single(zeros(1,1));  
        for i = 1:length(Px)   
            Pt = 1.05*sqrt(Px(i)^2 + Py(i)^2)/max(1,0.5*(TarEgoV(i) + vEgo));  %规划时间
            t_Vego = max(vEgo,1);
            t0 = single(0);
            tn = Pt;
            
            T = [t0^5,t0^4,t0^3,t0^2,t0,1;...
                5*t0^4,4*t0^3,3*t0^2,2*t0,1,0;...
                20*t0^3,12*t0^2,6*t0,2,0,0;...
                tn^5,tn^4,tn^3,tn^2,tn,1;...
                5*tn^4,4*tn^3,3*tn^2,2*tn,1,0;...
                20*tn^3,12*tn^2,6*tn,2,0,0];    
            
            Vn = TarEgoV(i);
            An = TarEgoAx(i);
            kP =  3*TarLineC3*(Px(i).^2) + 2*TarLineC2*Px(i) + TarLineC1;  %规划线的斜率
            
            Kap = 6*TarLineC3*(Px(i))+2*TarLineC2;      
            Arcf = (vEgo^2)*Kap;                          
            Ayn = Arcf/sqrt(1 + kP^2);                       
            Axn = Arcf*kP/sqrt(1 + kP^2);                              
            Vxn = Vn/sqrt(1 + kP^2);                         
            Vyn = Vn*kP/sqrt(1 + kP^2);
            
            MaX = [0;t_Vego;axEgo;Px(i);Vxn;Axn];            
            MaY = [0;0;(vEgo^2)*kapEgo;Py(i);Vyn;Ayn];
            %求解多项式
            A = T\MaX;
            B = T\MaY;
            
            a5 = A(1);
            a4 = A(2);
            a3 = A(3);
            a2 = A(4);
            a1 = A(5);
            a0 = A(6);
            
            b5 = B(1);
            b4 = B(2);
            b3 = B(3);
            b2 = B(4);
            b1 = B(5);
            b0 = B(6);
            
            preLineValid = true;
            for j=1:11
                t = (j-1)*tn/10;
                x(j) = a5*t^5 + a4*t^4 + a3*t^3 + a2*t^2 + a1*t + a0;
                Vx(j) = 5*a5*t^4 + 4*a4*t^3 + 3*a3*t^2 + 2*a2*t + a1;
                Ax(j) = 20*a5*t^3 + 12*a4*t^2 + 6*a3*t + 2*a2;
                y(j) = b5*t^5 + b4*t^4 + b3*t^3 + b2*t^2 + b1*t + b0;
                Vy(j) = 5*b5*t^4 + 4*b4*t^3 + 3*b3*t^2 + 2*b2*t + b1;
                Ay(j) = 20*b5*t^3 + 12*b4*t^2 + 6*b3*t + 2*b2;
                AyDt(j) = 60*b5*t^2 + 24*b4*t + 6*b3;

                if (abs(AyDt(j))>ayDtLimit)
                    break_Flg = uint8(1);
                    break_AyValue = abs(Ay(j));
                    break_AyDtValue = abs(AyDt(j));
                    preLineValid = false;
                    break;
                end
            end
            if ((sqrt(x(11)^2 + y(11)^2)) < Min_PlanDis) || ((sqrt(x(11)^2 + y(11)^2))*Dis_Fac < (PreDis + 2.1))
                preLineValid = false;
            end
            if preLineValid
                break_Flg = uint8(3);
                break_AyValue = max(abs(Ay));
                break_AyDtValue = max(abs(AyDt(j)));
                break;
            end
            
            if i == length(Px) % 此处存在都不满足的情况，需要按最长时间输出。经测试发现如果按最长时间输出会控不住车辆。暂时改成跟随目标线
                planValid = true;
                Pt = single(Px(i));
                x = single(zeros(11,1));
                y = single(zeros(11,1));
                x = single((linspace(0,40,11)))';
                y = TarLineC3.*x.^3 + TarLineC2.*x.^2 + TarLineC1*x + TarLineC0;
                break_Flg = uint8(4);
                break_AyValue = single(0);
                break_AyDtValue = single(0);
            end
        end
        LoopNum = i;
        planValid = true;
        planT = Pt;
        planX = x;
        planY = y;
        planLength = planX(end,1);
    end
else
    planValid = false;
    planT = single(0);
    planX = single(zeros(11,1));
    planY = single(zeros(11,1));
    LoopNum = 0;
    planLength = planX(end,1);
    Ay = single(zeros(11,1));
    AyDt = single(zeros(11,1));
    break_Flg = uint8(0);
    break_AyValue = single(0);
    break_AyDtValue = single(0);
end

== matlab function PvtSubSys_LATC/Subsystem/LateralControl/LCS_Angle/Motion_Planning/FrenetTrajectory/Subsystem/MATLAB Function1 ==
  data: Delaytime input uint16; Flg output uint8; Count output uint16; TarDangerLevel input uint8; TarDangerLevelK1 input uint8; FlgK1 input uint8; CountK1 input uint16
function [Flg,Count]= fcn(Delaytime,TarDangerLevel,TarDangerLevelK1,FlgK1,CountK1)
Count = min(CountK1 + uint16(1),Delaytime);
if Count == Delaytime
    Flg = uint8(0);
else
    Flg = FlgK1;
end
%%状态检测
if TarDangerLevel == uint8(1) && TarDangerLevelK1 == 0 %功能激活
    Count = uint16(0);
    Flg = uint8(1);  
end
end

== matlab function PvtSubSys_LATC/Subsystem/LateralControl/EPSFaultCheck/MATLAB Function1 ==
  data: u input; y output uint8; countK input uint8; count output uint8
function [y,count] = fcn(u,countK)
count = countK - uint8(1);
if u>0
    count = uint8(3000);
end
if count > 1
    y = uint8(0);
else
    y = uint8(1);
end
